simulink library "lib_fuel_converter3"  (Simulink 4.1.1)
values from neighbouring files (symbols this model uses):
  logFlag = 1    [advSACompMaskInit.m]    (also in advSACompMaskInitR13.m)
undefined symbols (not defined in the file or in its folder): air_cp, amb_tmp, cyc_mph, ex_gas_cp, fc_acc_mass, fc_base_mass, fc_c2i_th_cond, fc_c_init_tmp, fc_cl2h_eff, fc_CO2_to_FUELgps, fc_cold, fc_cold_tmp, fc_cp, fc_ct_trq, fc_emisv, fc_ext_sarea, fc_fuel_den, fc_fuel_lhv, fc_h2x_th_cond, fc_h_air_flow, fc_h_cp, fc_h_init_tmp, fc_hood_emisv, fc_hood_sarea, fc_i2x_th_cond, fc_i_init_tmp, fc_inertia, fc_map_spd, fc_map_trq, fc_max_trq, fc_nn_model_name, fc_pwr_scale, fc_spd_scale, fc_trq_scale, fc_tstat, fc_x_init_tmp, fd_ratio, gb_num_init, gb_ratio, generalName, pow, vc_idle_bool, vc_idle_spd, vc_key_on, veh_glider_mass, wh_radius
libraries: lib_fuel_converter3 x4, lib_etc x4, lib_fuel_converter x2, lib_fuel_converter2 x1
(part 7 of 9)

== system lib_fuel_converter3/fuel converter <fc> no fuel at negative torque/IC Engine Model  &  Interface/ic engine model/requested power and energy ==
  trq : Inport  Port=1  LatchInput=off
  spd : Inport  Port=2  LatchInput=off
  Integrator : Integrator  ExternalReset=none  InitialConditionSource=internal  InitialCondition=0  LimitOutput=off  UpperSaturationLimit=inf  LowerSaturationLimit=-inf  ShowSaturationPort=off  ShowStatePort=off  AbsoluteTolerance=auto
  J : Subsystem  TreatAsAtomicUnit=on  mask(enhancedToWorkspace){generalName=generalName, specificName=energy_r, logFlag=logFlag}
      mask prompts: generalName "General Name [char-evaluated]"; specificName "Specific Name [char-literal]"; logFlag "Enable flag (1=on,0=off)"
      mask help: A wrapper for the Simulink "To Workspace" block that allows you to evaluate the name of the variable to log to workspace. This is useful to avoid the double logging errors that occur when you pull in two library models that attempt to log to the same variable.
      mask init:
      | enhancedToWsMaker
      settings: CopyFcn=breakLinkCopyFcn  ParentCloseFcn=breakLinkParCloseFcn  RTWFcnNameOpts=Auto  RTWFileNameOpts=Auto
      mask Help:
      | <h2>Enhanced To Workspace Block</h2>
      | <h3>Parameters</h3>
      | <UL>
      | <li><b>General Name:</b> This is the more general name of the variable. Variables are saved to the workspace as <i>generalName_specificName</i>. Note that this is an evaluated variable. If you would like to type in the value directly, it must be surrounded with single quotes. Otherwise you can input the name of a variable containing a char string.</li>
      | <li><b>Specific Name:</b> This is the specific name of the variable. Note that this is input as a char literal (i.e., you don't need quotes).</li>
      | <li><b>Enable Flag:</b> This flag should have the value of 0 or 1. If 0, the variable will not be logged to the workspace. If 1, the variable will be logged. This is done so that variable logging can be turned off to improve speed.</li>
      | </ul>
      | <h3>Overview</h3>
      | <p>The enhanced to workspace block was put together to allow one to dynamically resolve variable names at run time in simulink. This is most powerful when used in conjunction with a masked subsystem to allow multiple instances of that masked subsytem to be used in the same model. The strategy is to set the generalName in the block mask which will allow the block to change the general name for all variable logging on the fly.
      | <h3>Helper Files</h3>
      | <p>Three m-files are required by the enhancedToWorkspace block. These files are located in the &lt; ADVISOR root &gt;/GUI directory :
      | <ul>
      | <li><i>enhancedToWsMaker.m</i> This file runs the mask initialization for the block</li>
      | <li><i>breakLinkCopyFcn.m</i> This file is used by the block callback when the simulink block is copied. It is necessary to break the link to the enhancedToWorkspace similar to the To Workspace block in order for it to be able to configure itself. (Try copying simulink's To Workspace block--it is impossible to make a link)</li>
      | <li><i>breakLinkParCloseFcn.m</i> This file is similar to the breakLinkCopyFcn and is used when a parent system is closed</li>
      | </ul>
      | <hr>
      | 
      | <p>Created 2003-Jan-21, Michael Patrick O'Keefe, NREL</p>
      | 
      | <!--
      | <VARDEF>
      | <H3>var_name</H3>
      | <UL>
      | <LI><B>data type</B> data type here</LI>
      | <LI><B>units</B> units here</LI>
      | <LI><B>vehicle type</B> vehicle type here</LI>
      | <LI><B>description</B> description here</LI>
      | </UL>
      | </VARDEF>
      | -->
      mask Display: disp([generalName,'_',specificName])
  Product : Product  Inputs=2  Multiplication=Element-wise(.*)  SaturateOnIntegerOverflow=on
  hp : Subsystem  TreatAsAtomicUnit=on  mask(enhancedToWorkspace){generalName=generalName, specificName=pwr_r_hp, logFlag=logFlag}
      mask prompts: generalName "General Name [char-evaluated]"; specificName "Specific Name [char-literal]"; logFlag "Enable flag (1=on,0=off)"
      mask help: A wrapper for the Simulink "To Workspace" block that allows you to evaluate the name of the variable to log to workspace. This is useful to avoid the double logging errors that occur when you pull in two library models that attempt to log to the same variable.
      mask init:
      | enhancedToWsMaker
      settings: CopyFcn=breakLinkCopyFcn  ParentCloseFcn=breakLinkParCloseFcn  RTWFcnNameOpts=Auto  RTWFileNameOpts=Auto
      mask Help:
      | <h2>Enhanced To Workspace Block</h2>
      | <h3>Parameters</h3>
      | <UL>
      | <li><b>General Name:</b> This is the more general name of the variable. Variables are saved to the workspace as <i>generalName_specificName</i>. Note that this is an evaluated variable. If you would like to type in the value directly, it must be surrounded with single quotes. Otherwise you can input the name of a variable containing a char string.</li>
      | <li><b>Specific Name:</b> This is the specific name of the variable. Note that this is input as a char literal (i.e., you don't need quotes).</li>
      | <li><b>Enable Flag:</b> This flag should have the value of 0 or 1. If 0, the variable will not be logged to the workspace. If 1, the variable will be logged. This is done so that variable logging can be turned off to improve speed.</li>
      | </ul>
      | <h3>Overview</h3>
      | <p>The enhanced to workspace block was put together to allow one to dynamically resolve variable names at run time in simulink. This is most powerful when used in conjunction with a masked subsystem to allow multiple instances of that masked subsytem to be used in the same model. The strategy is to set the generalName in the block mask which will allow the block to change the general name for all variable logging on the fly.
      | <h3>Helper Files</h3>
      | <p>Three m-files are required by the enhancedToWorkspace block. These files are located in the &lt; ADVISOR root &gt;/GUI directory :
      | <ul>
      | <li><i>enhancedToWsMaker.m</i> This file runs the mask initialization for the block</li>
      | <li><i>breakLinkCopyFcn.m</i> This file is used by the block callback when the simulink block is copied. It is necessary to break the link to the enhancedToWorkspace similar to the To Workspace block in order for it to be able to configure itself. (Try copying simulink's To Workspace block--it is impossible to make a link)</li>
      | <li><i>breakLinkParCloseFcn.m</i> This file is similar to the breakLinkCopyFcn and is used when a parent system is closed</li>
      | </ul>
      | <hr>
      | 
      | <p>Created 2003-Jan-21, Michael Patrick O'Keefe, NREL</p>
      | 
      | <!--
      | <VARDEF>
      | <H3>var_name</H3>
      | <UL>
      | <LI><B>data type</B> data type here</LI>
      | <LI><B>units</B> units here</LI>
      | <LI><B>vehicle type</B> vehicle type here</LI>
      | <LI><B>description</B> description here</LI>
      | </UL>
      | </VARDEF>
      | -->
      mask Display: disp([generalName,'_',specificName])
  "w -> hp" : Gain  Gain=0.001341022  Multiplication=Element-wise(K.*u)  SaturateOnIntegerOverflow=on
  watts : Subsystem  TreatAsAtomicUnit=on  mask(enhancedToWorkspace){generalName=generalName, specificName=pwr_r, logFlag=logFlag}
      mask prompts: generalName "General Name [char-evaluated]"; specificName "Specific Name [char-literal]"; logFlag "Enable flag (1=on,0=off)"
      mask help: A wrapper for the Simulink "To Workspace" block that allows you to evaluate the name of the variable to log to workspace. This is useful to avoid the double logging errors that occur when you pull in two library models that attempt to log to the same variable.
      mask init:
      | enhancedToWsMaker
      settings: CopyFcn=breakLinkCopyFcn  ParentCloseFcn=breakLinkParCloseFcn  RTWFcnNameOpts=Auto  RTWFileNameOpts=Auto
      mask Help:
      | <h2>Enhanced To Workspace Block</h2>
      | <h3>Parameters</h3>
      | <UL>
      | <li><b>General Name:</b> This is the more general name of the variable. Variables are saved to the workspace as <i>generalName_specificName</i>. Note that this is an evaluated variable. If you would like to type in the value directly, it must be surrounded with single quotes. Otherwise you can input the name of a variable containing a char string.</li>
      | <li><b>Specific Name:</b> This is the specific name of the variable. Note that this is input as a char literal (i.e., you don't need quotes).</li>
      | <li><b>Enable Flag:</b> This flag should have the value of 0 or 1. If 0, the variable will not be logged to the workspace. If 1, the variable will be logged. This is done so that variable logging can be turned off to improve speed.</li>
      | </ul>
      | <h3>Overview</h3>
      | <p>The enhanced to workspace block was put together to allow one to dynamically resolve variable names at run time in simulink. This is most powerful when used in conjunction with a masked subsystem to allow multiple instances of that masked subsytem to be used in the same model. The strategy is to set the generalName in the block mask which will allow the block to change the general name for all variable logging on the fly.
      | <h3>Helper Files</h3>
      | <p>Three m-files are required by the enhancedToWorkspace block. These files are located in the &lt; ADVISOR root &gt;/GUI directory :
      | <ul>
      | <li><i>enhancedToWsMaker.m</i> This file runs the mask initialization for the block</li>
      | <li><i>breakLinkCopyFcn.m</i> This file is used by the block callback when the simulink block is copied. It is necessary to break the link to the enhancedToWorkspace similar to the To Workspace block in order for it to be able to configure itself. (Try copying simulink's To Workspace block--it is impossible to make a link)</li>
      | <li><i>breakLinkParCloseFcn.m</i> This file is similar to the breakLinkCopyFcn and is used when a parent system is closed</li>
      | </ul>
      | <hr>
      | 
      | <p>Created 2003-Jan-21, Michael Patrick O'Keefe, NREL</p>
      | 
      | <!--
      | <VARDEF>
      | <H3>var_name</H3>
      | <UL>
      | <LI><B>data type</B> data type here</LI>
      | <LI><B>units</B> units here</LI>
      | <LI><B>vehicle type</B> vehicle type here</LI>
      | <LI><B>description</B> description here</LI>
      | </UL>
      | </VARDEF>
      | -->
      mask Display: disp([generalName,'_',specificName])
  wires:
  "w -> hp"/1 -> hp/1(In1)
  Product/1 -> "w -> hp"/1, Integrator/1, watts/1(In1)
  Integrator/1 -> J/1(In1)
  trq/1 -> Product/1
  spd/1 -> Product/2

== system lib_fuel_converter3/Fuel Converter Control/Fuel Converter Control conventional ic engine/conventional IC engine/Fuel Converter Control/key_on ==
  Clock : Clock
      settings: DisplayTime=off  Decimation=10
  Fcn1 : Fcn  Expr=rem(u[1],period)
  Look-Up Table : Lookup  InputValues=t  OutputValues=y
  out_1 : Outport  Port=1  InitialOutput=0
  wires:
  Fcn1/1 -> Look-Up Table/1
  Clock/1 -> Fcn1/1
  Look-Up Table/1 -> out_1/1

== system lib_fuel_converter3/configurable subsystems/fuel use and EO emis/fc temp/fc mass heat flow/Block NOTES ==
  note: FUEL CONVERTER MASS HEAT LOSS
      | This block models the heat loss from a fuel converter (such as an IC engine).
      | Convection (as a function of vehicle speed), radiation, and conduction effects are included.
      | Engine cylinder (c), interior (i), exterior (x) and hood (h)
      | heat flows are estimated based on the temperatures from the previous iteration.

== system lib_fuel_converter3/configurable subsystems/fuel use and EO emis/fc temp/old fc coolant  temp. (C)/Block NOTES ==
  note: This block computes engine coolant temperature,
      | assuming that it asymptotically approaches its maximum
      | temperature when the engine is on, and asymptotically
      | approaches the ambient temperature when the engine
      | is off.  Temperatue rise rate is assumed to be a function
      | only of current engine coolant temperature, and the fall
      | rate is also a function of vehicle speed and ambient temperature.
      | There is no dependence on engine load or speed.

== system lib_fuel_converter3/configurable subsystems/fuel use and EO emis/fc temp correct/fc temp correct Constant Correction Factors (Equation Based)/Block NOTES ==
  note: This block determines actual fuel use and engine-out emissions
      | given the fully hot values and the engine coolant temperature.
      | The correlations used here were developed at NREL using
      | Hot and Cold Engine data collected
      | at Oak Ridge National Laboratory.

== system lib_fuel_converter3/configurable subsystems/fuel use and EO emis/fc temp correct/fc temp correct Variable Correction Factors (Map Based)/CO factor cold-to-hot ==
  x0 : Inport  Port=1  LatchInput=off
  y0 : Inport  Port=2  LatchInput=off
  Mux : Mux  Inputs=2
      settings: DisplayOption=none
  S-function : S-Function  FunctionName=sftable2  Parameters=xindex, yindex, table  PortCounts=[]  SFunctionModules=''
  table out : Outport  Port=1  InitialOutput=0
  wires:
  y0/1 -> Mux/2
  S-function/1 -> table out/1
  x0/1 -> Mux/1
  Mux/1 -> S-function/1

== system lib_fuel_converter3/configurable subsystems/fuel use and EO emis/fc temp correct/fc temp correct Variable Correction Factors (Map Based)/HC factor cold-to-hot ==
  x0 : Inport  Port=1  LatchInput=off
  y0 : Inport  Port=2  LatchInput=off
  Mux : Mux  Inputs=2
      settings: DisplayOption=none
  S-function : S-Function  FunctionName=sftable2  Parameters=xindex, yindex, table  PortCounts=[]  SFunctionModules=''
  table out : Outport  Port=1  InitialOutput=0
  wires:
  y0/1 -> Mux/2
  S-function/1 -> table out/1
  x0/1 -> Mux/1
  Mux/1 -> S-function/1

== system lib_fuel_converter3/configurable subsystems/fuel use and EO emis/fc temp correct/fc temp correct Variable Correction Factors (Map Based)/NOx factor cold-to-hot ==
  x0 : Inport  Port=1  LatchInput=off
  y0 : Inport  Port=2  LatchInput=off
  Mux : Mux  Inputs=2
      settings: DisplayOption=none
  S-function : S-Function  FunctionName=sftable2  Parameters=xindex, yindex, table  PortCounts=[]  SFunctionModules=''
  table out : Outport  Port=1  InitialOutput=0
  wires:
  y0/1 -> Mux/2
  S-function/1 -> table out/1
  x0/1 -> Mux/1
  Mux/1 -> S-function/1

== system lib_fuel_converter3/configurable subsystems/fuel use and EO emis/fc temp correct/fc temp correct Variable Correction Factors (Map Based)/PM factor cold-to-hot ==
  x0 : Inport  Port=1  LatchInput=off
  y0 : Inport  Port=2  LatchInput=off
  Mux : Mux  Inputs=2
      settings: DisplayOption=none
  S-function : S-Function  FunctionName=sftable2  Parameters=xindex, yindex, table  PortCounts=[]  SFunctionModules=''
  table out : Outport  Port=1  InitialOutput=0
  wires:
  y0/1 -> Mux/2
  S-function/1 -> table out/1
  x0/1 -> Mux/1
  Mux/1 -> S-function/1

== system lib_fuel_converter3/configurable subsystems/fuel use and EO emis/fc temp correct/fc temp correct Variable Correction Factors (Map Based)/fuel factor cold-to-hot ==
  x0 : Inport  Port=1  LatchInput=off
  y0 : Inport  Port=2  LatchInput=off
  Mux : Mux  Inputs=2
      settings: DisplayOption=none
  S-function : S-Function  FunctionName=sftable2  Parameters=xindex, yindex, table  PortCounts=[]  SFunctionModules=''
  table out : Outport  Port=1  InitialOutput=0
  wires:
  y0/1 -> Mux/2
  S-function/1 -> table out/1
  x0/1 -> Mux/1
  Mux/1 -> S-function/1

== system lib_fuel_converter3/configurable subsystems/fuel use and EO emis Neural Network Model/fc temp/fc mass heat flow/Block NOTES ==
  note: FUEL CONVERTER MASS HEAT LOSS
      | This block models the heat loss from a fuel converter (such as an IC engine).
      | Convection (as a function of vehicle speed), radiation, and conduction effects are included.
      | Engine cylinder (c), interior (i), exterior (x) and hood (h)
      | heat flows are estimated based on the temperatures from the previous iteration.

== system lib_fuel_converter3/configurable subsystems/fuel use and EO emis Neural Network Model/fc temp/old fc coolant  temp. (C)/Block NOTES ==
  note: This block computes engine coolant temperature,
      | assuming that it asymptotically approaches its maximum
      | temperature when the engine is on, and asymptotically
      | approaches the ambient temperature when the engine
      | is off.  Temperatue rise rate is assumed to be a function
      | only of current engine coolant temperature, and the fall
      | rate is also a function of vehicle speed and ambient temperature.
      | There is no dependence on engine load or speed.

== system lib_fuel_converter3/configurable subsystems/fuel use and EO emis Neural Network Model/fc temp correct/fc temp correct Constant Correction Factors (Equation Based)/Block NOTES ==
  note: This block determines actual fuel use and engine-out emissions
      | given the fully hot values and the engine coolant temperature.
      | The correlations used here were developed at NREL using
      | Hot and Cold Engine data collected
      | at Oak Ridge National Laboratory.

== system lib_fuel_converter3/configurable subsystems/fuel use and EO emis Neural Network Model/fc temp correct/fc temp correct Variable Correction Factors (Map Based)/CO factor cold-to-hot ==
  x0 : Inport  Port=1  LatchInput=off
  y0 : Inport  Port=2  LatchInput=off
  Mux : Mux  Inputs=2
      settings: DisplayOption=none
  S-function : S-Function  FunctionName=sftable2  Parameters=xindex, yindex, table  PortCounts=[]  SFunctionModules=''
  table out : Outport  Port=1  InitialOutput=0
  wires:
  y0/1 -> Mux/2
  S-function/1 -> table out/1
  x0/1 -> Mux/1
  Mux/1 -> S-function/1

== system lib_fuel_converter3/configurable subsystems/fuel use and EO emis Neural Network Model/fc temp correct/fc temp correct Variable Correction Factors (Map Based)/HC factor cold-to-hot ==
  x0 : Inport  Port=1  LatchInput=off
  y0 : Inport  Port=2  LatchInput=off
  Mux : Mux  Inputs=2
      settings: DisplayOption=none
  S-function : S-Function  FunctionName=sftable2  Parameters=xindex, yindex, table  PortCounts=[]  SFunctionModules=''
  table out : Outport  Port=1  InitialOutput=0
  wires:
  y0/1 -> Mux/2
  S-function/1 -> table out/1
  x0/1 -> Mux/1
  Mux/1 -> S-function/1

== system lib_fuel_converter3/configurable subsystems/fuel use and EO emis Neural Network Model/fc temp correct/fc temp correct Variable Correction Factors (Map Based)/NOx factor cold-to-hot ==
  x0 : Inport  Port=1  LatchInput=off
  y0 : Inport  Port=2  LatchInput=off
  Mux : Mux  Inputs=2
      settings: DisplayOption=none
  S-function : S-Function  FunctionName=sftable2  Parameters=xindex, yindex, table  PortCounts=[]  SFunctionModules=''
  table out : Outport  Port=1  InitialOutput=0
  wires:
  y0/1 -> Mux/2
  S-function/1 -> table out/1
  x0/1 -> Mux/1
  Mux/1 -> S-function/1

== system lib_fuel_converter3/configurable subsystems/fuel use and EO emis Neural Network Model/fc temp correct/fc temp correct Variable Correction Factors (Map Based)/PM factor cold-to-hot ==
  x0 : Inport  Port=1  LatchInput=off
  y0 : Inport  Port=2  LatchInput=off
  Mux : Mux  Inputs=2
      settings: DisplayOption=none
  S-function : S-Function  FunctionName=sftable2  Parameters=xindex, yindex, table  PortCounts=[]  SFunctionModules=''
  table out : Outport  Port=1  InitialOutput=0
  wires:
  y0/1 -> Mux/2
  S-function/1 -> table out/1
  x0/1 -> Mux/1
  Mux/1 -> S-function/1

== system lib_fuel_converter3/configurable subsystems/fuel use and EO emis Neural Network Model/fc temp correct/fc temp correct Variable Correction Factors (Map Based)/fuel factor cold-to-hot ==
  x0 : Inport  Port=1  LatchInput=off
  y0 : Inport  Port=2  LatchInput=off
  Mux : Mux  Inputs=2
      settings: DisplayOption=none
  S-function : S-Function  FunctionName=sftable2  Parameters=xindex, yindex, table  PortCounts=[]  SFunctionModules=''
  table out : Outport  Port=1  InitialOutput=0
  wires:
  y0/1 -> Mux/2
  S-function/1 -> table out/1
  x0/1 -> Mux/1
  Mux/1 -> S-function/1

== system lib_fuel_converter3/fuel converter  <fc> for series/Model & Interface/model/providing trq (+ive or -ive)/effect of inertia (Nm) ==
  note: if initial speed is >0 and it is the
      | first time step ignore inertial loads
      | tm:2/6/01
  req'd spd (rad/s) : Inport  Port=1  LatchInput=off
  prev spd : Inport  Port=2  LatchInput=off
  Clock : Clock
      settings: DisplayTime=off  Decimation=10
  Constant : Constant  Value=fc_inertia
  Constant1 : Constant  Value=cyc_mph(1,2)
  Logical Operator : Logic  Operator=NAND  Inputs=2
  Logical Operator1 : Logic  Operator=NOT  Inputs=2
  Memory : Memory  X0=-0.1  InheritSampleTime=off
      settings: RTWStateStorageClass=Auto
  Memory1 : Memory  X0=0  InheritSampleTime=off
      settings: RTWStateStorageClass=Auto
  Product1 : Product  Inputs=**/*  Multiplication=Element-wise(.*)  SaturateOnIntegerOverflow=on
  Sum : Sum  Inputs=+-  SaturateOnIntegerOverflow=on
  Sum1 : Sum  Inputs=+-  SaturateOnIntegerOverflow=on
  (Nm) : Outport  Port=1  InitialOutput=0
  wires:
  Logical Operator1/1 -> Logical Operator/2
  Memory1/1 -> Logical Operator1/1
  Constant1/1 -> Logical Operator/1
  Logical Operator/1 -> Product1/4
  Sum/1 -> Product1/2
  Sum1/1 -> Product1/3
  req'd spd (rad/s)/1 -> Sum/1
  prev spd/1 -> Sum/2
  Product1/1 -> (Nm)/1
  Memory/1 -> Sum1/2
  Clock/1 -> Memory1/1, Memory/1, Sum1/1
  Constant/1 -> Product1/1

== system lib_fuel_converter3/fuel converter  <fc> for series/Model & Interface/model/providing trq (+ive or -ive)/enforce engine limits ==
  req'd engine trq (Nm) : Inport  Port=1  LatchInput=off
  req'd engine spd (rad/s) : Inport  Port=2  LatchInput=off
  Block NOTES : Subsystem
      settings: RTWFcnNameOpts=Auto  RTWFileNameOpts=Auto
      mask Display: disp('Block\nNOTES')
  MinMax : MinMax  Function=min  Inputs=2
  MinMax1 : MinMax  Function=max  Inputs=2
  Relational Operator : RelationalOperator  Operator=~=
  Saturation : Saturate  UpperLimit=max(fc_map_spd)*fc_spd_scale  LowerLimit=0  LinearizeAsGain=on
  T_closed throttle : lib_fuel_converter/fuel converter  <fc> for series/providing trq (+ive or -ive)/enforce engine limits/T_closed throttle
      settings: RTWFcnNameOpts=Auto  RTWFileNameOpts=Auto
  T_max : Subsystem
      settings: RTWFcnNameOpts=Auto  RTWFileNameOpts=Auto
  clutch disengaged1 : RelationalOperator  Operator=~=
  limited engine brake trq (Nm) : Outport  Port=1
  limited engine spd (rad/s) : Outport  Port=2
  tag scope: fc_spd_limited=scoped, fc_trq_limited=scoped
  wires:
  Relational Operator/1 -> [fc_spd_limited]
  MinMax/1 -> MinMax1/1
  T_max/1(T_max) -> MinMax/2
  clutch disengaged1/1 -> [fc_trq_limited]
  MinMax1/1 -> limited engine brake trq (Nm)/1, clutch disengaged1/2
  req'd engine trq (Nm)/1 -> MinMax/1, clutch disengaged1/1
  Saturation/1 -> T_closed throttle/1, T_max/1(w_APU), limited engine spd (rad/s)/1, Relational Operator/2
  req'd engine spd (rad/s)/1 -> Saturation/1, Relational Operator/1
  T_closed throttle/1 -> MinMax1/2

== system lib_fuel_converter3/fuel converter  <fc> for series/Model & Interface/model/spinning up or spinning down/T_closed throttle ==
  w_APU : Inport  Port=1  LatchInput=off
  Saturation : Saturate  UpperLimit=max(fc_map_spd)*fc_spd_scale  LowerLimit=min(fc_map_spd)*fc_spd_scale  LinearizeAsGain=on
  ctt lookup : Lookup  InputValues=fc_map_spd*fc_spd_scale  OutputValues=fc_ct_trq*fc_trq_scale
  T_closed throttle : Outport  Port=1  InitialOutput=0
  wires:
  w_APU/1 -> Saturation/1
  Saturation/1 -> ctt lookup/1
  ctt lookup/1 -> T_closed throttle/1

== system lib_fuel_converter3/fuel converter  <fc> for series/Model & Interface/model/spinning up or spinning down/T_max ==
  w_APU : Inport  Port=1  LatchInput=off
  Saturation1 : Saturate  UpperLimit=max(fc_map_spd)*fc_spd_scale  LowerLimit=min(fc_map_spd)*fc_spd_scale  LinearizeAsGain=on
  max_torque lookup : Lookup  InputValues=fc_map_spd*fc_spd_scale  OutputValues=fc_max_trq*fc_trq_scale
  T_max : Outport  Port=1  InitialOutput=0
  wires:
  max_torque lookup/1 -> T_max/1
  w_APU/1 -> Saturation1/1
  Saturation1/1 -> max_torque lookup/1

== system lib_fuel_converter3/fuel converter  <fc> for series/Model & Interface/model/spinning up or spinning down/dt ==
  Clock : Clock
      settings: DisplayTime=off  Decimation=10
  Memory1 : Memory  X0=-0.1  InheritSampleTime=off
      settings: RTWStateStorageClass=Auto
  Sum1 : Sum  Inputs=+-  SaturateOnIntegerOverflow=on
  out_1 : Outport  Port=1  InitialOutput=0
  wires:
  Sum1/1 -> out_1/1
  Memory1/1 -> Sum1/2
  Clock/1 -> Memory1/1, Sum1/1

== system lib_fuel_converter3/fuel converter  <fc> for series/Model & Interface/model/spinning up or spinning down/effect of inertia (Nm) ==
  note: if initial speed is >0 and it is the
      | first time step ignore inertial loads
      | tm:2/6/01
  req'd spd (rad/s) : Inport  Port=1  LatchInput=off
  prev spd : Inport  Port=2  LatchInput=off
  Clock : Clock
      settings: DisplayTime=off  Decimation=10
  Constant : Constant  Value=fc_inertia
  Constant1 : Constant  Value=cyc_mph(1,2)
  Logical Operator : Logic  Operator=NAND  Inputs=2
  Logical Operator1 : Logic  Operator=NOT  Inputs=2
  Memory : Memory  X0=-0.1  InheritSampleTime=off
      settings: RTWStateStorageClass=Auto
  Memory1 : Memory  X0=0  InheritSampleTime=off
      settings: RTWStateStorageClass=Auto
  Product1 : Product  Inputs=**/*  Multiplication=Element-wise(.*)  SaturateOnIntegerOverflow=on
  Sum : Sum  Inputs=+-  SaturateOnIntegerOverflow=on
  Sum1 : Sum  Inputs=+-  SaturateOnIntegerOverflow=on
  (Nm) : Outport  Port=1  InitialOutput=0
  wires:
  Constant/1 -> Product1/1
  Clock/1 -> Sum1/1, Memory/1, Memory1/1
  Memory/1 -> Sum1/2
  Product1/1 -> (Nm)/1
  prev spd/1 -> Sum/2
  req'd spd (rad/s)/1 -> Sum/1
  Sum1/1 -> Product1/3
  Sum/1 -> Product1/2
  Logical Operator/1 -> Product1/4
  Constant1/1 -> Logical Operator/1
  Memory1/1 -> Logical Operator1/1
  Logical Operator1/1 -> Logical Operator/2

== system lib_fuel_converter3/fuel converter  <fc> for series/Model & Interface/model/spinning up or spinning down/just started spin-down/spin-up ==
  state : Inport  Port=1  LatchInput=off
  Logical Operator : Logic  Operator=AND  Inputs=2
  Logical Operator1 : Logic  Operator=NOT  Inputs=1
  Memory1 : Memory  X0=(cyc_mph(1,2)==0)  InheritSampleTime=off
      settings: RTWStateStorageClass=Auto
  trigger : Outport  Port=1  InitialOutput=0
  wires:
  state/1 -> Memory1/1, Logical Operator/1
  Logical Operator/1 -> trigger/1
  Logical Operator1/1 -> Logical Operator/2
  Memory1/1 -> Logical Operator1/1

== system lib_fuel_converter3/fuel converter  <fc> for series/Model & Interface/model/spinning up or spinning down/no-lag Reset Integrator ==
  in_1 : Inport  Port=1  LatchInput=off
  in_2 : Inport  Port=2  LatchInput=off
  in_3 : Inport  Port=3  LatchInput=off
  Constant : Constant  Value=0
  Memory : Memory  Orientation=left  X0=initval  InheritSampleTime=off
      settings: RTWStateStorageClass=Auto
  Product : Product  Inputs=2  Multiplication=Element-wise(.*)  SaturateOnIntegerOverflow=on
  Sum : Sum  Inputs=++  SaturateOnIntegerOverflow=on
  Switch : Switch  Threshold=eps
  dt : lib_fuel_converter/fuel converter  <fc> for series/spinning up or spinning down/no-lag Reset Integrator/dt  Orientation=down
      settings: RTWFcnNameOpts=Auto  RTWFileNameOpts=Auto
  in_2==0 : RelationalOperator  Operator===
  out_1 : Outport  Port=1  InitialOutput=0
  wires:
  Constant/1 -> in_2==0/2
  in_2==0/1 -> Switch/2
  Switch/1 -> Memory/1, out_1/1
  Sum/1 -> Switch/1
  Memory/1 -> Sum/1
  Product/1 -> Sum/2
  dt/1 -> Product/1
  in_1/1 -> Product/2
  in_2/1 -> in_2==0/1
  in_3/1 -> Switch/3

== system lib_fuel_converter3/fuel converter <fc>/IC Engine Model  &  Interface/ic engine model/engine speed estimator/Block NOTES ==
  note: If the clutch is engaged and the trace was missed in the previous time step:
      | The estimated engine speed for the current time step is the actual engine
      | speed from the previous time step.
      |
      | If the clutch is disengaged and the speed is commanded to increase (spin up):
      | The engine speed is the lesser of the commanded speed and the maximum
      | speed attainable given the engine capability.
      |
      | If the clutch is disengaged at the speed is commanded to decrease (spin down):
      | The engine speed is computed by integrating with respect to time the ratio of
      |  closed-throttle torque to engine inertia.
      |
      | Otherwise:
      | The engine speed is equal to the speed command, but no greater than the
      | engine's maximum speed nor less than the engine's idle speed (if the engine is on.)

== system lib_fuel_converter3/fuel converter <fc>/IC Engine Model  &  Interface/ic engine model/engine speed estimator/dt ==
  Clock : Clock
      settings: DisplayTime=off  Decimation=10
  Memory1 : Memory  X0=-0.1  InheritSampleTime=off
      settings: RTWStateStorageClass=Auto
  Sum1 : Sum  Inputs=+-  SaturateOnIntegerOverflow=on
  out_1 : Outport  Port=1  InitialOutput=0
  wires:
  Sum1/1 -> out_1/1
  Memory1/1 -> Sum1/2
  Clock/1 -> Memory1/1, Sum1/1

== system lib_fuel_converter3/fuel converter <fc>/IC Engine Model  &  Interface/ic engine model/engine speed estimator/effect of inertia (Nm) ==
  req'd spd (rad/s) : Inport  Port=1  LatchInput=off
  prev spd : Inport  Port=2  LatchInput=off
  Clock : Clock
      settings: DisplayTime=off  Decimation=10
  Constant : Constant  Value=fc_inertia
  Memory : Memory  X0=-0.1  InheritSampleTime=off
      settings: RTWStateStorageClass=Auto
  Product1 : Product  Inputs=**/  Multiplication=Element-wise(.*)  SaturateOnIntegerOverflow=on
  Sum : Sum  Inputs=+-  SaturateOnIntegerOverflow=on
  Sum1 : Sum  Inputs=+-  SaturateOnIntegerOverflow=on
  (Nm) : Outport  Port=1  InitialOutput=0
  wires:
  Sum/1 -> Product1/2
  Sum1/1 -> Product1/3
  req'd spd (rad/s)/1 -> Sum/1
  prev spd/1 -> Sum/2
  Product1/1 -> (Nm)/1
  Memory/1 -> Sum1/2
  Clock/1 -> Memory/1, Sum1/1
  Constant/1 -> Product1/1

== system lib_fuel_converter3/fuel converter <fc>/IC Engine Model  &  Interface/ic engine model/engine speed estimator/just started spin-down/spin-up ==
  state : Inport  Port=1  LatchInput=off
  Logical Operator : Logic  Operator=AND  Inputs=2
  Logical Operator1 : Logic  Operator=NOT  Inputs=1
  Memory1 : Memory  X0=1  InheritSampleTime=off
      settings: RTWStateStorageClass=Auto
  trigger : Outport  Port=1  InitialOutput=0
  wires:
  Memory1/1 -> Logical Operator1/1
  Logical Operator1/1 -> Logical Operator/2
  Logical Operator/1 -> trigger/1
  state/1 -> Logical Operator/1, Memory1/1

== system lib_fuel_converter3/fuel converter <fc>/IC Engine Model  &  Interface/ic engine model/engine speed estimator/no-lag Reset Integrator ==
  in_1 : Inport  Port=1  LatchInput=off
  in_2 : Inport  Port=2  LatchInput=off
  in_3 : Inport  Port=3  LatchInput=off
  Constant : Constant  Value=0
  Memory : Memory  Orientation=left  X0=initval  InheritSampleTime=off
      settings: RTWStateStorageClass=Auto
  Product : Product  Inputs=2  Multiplication=Element-wise(.*)  SaturateOnIntegerOverflow=on
  Sum : Sum  Inputs=++  SaturateOnIntegerOverflow=on
  Switch : Switch  Threshold=eps
  dt : Subsystem  Orientation=down
      settings: RTWFcnNameOpts=Auto  RTWFileNameOpts=Auto
  in_2==0 : RelationalOperator  Operator===
  out_1 : Outport  Port=1  InitialOutput=0
  wires:
  in_3/1 -> Switch/3
  in_2/1 -> in_2==0/1
  in_1/1 -> Product/2
  dt/1(out_1) -> Product/1
  Product/1 -> Sum/2
  Memory/1 -> Sum/1
  Sum/1 -> Switch/1
  Switch/1 -> out_1/1, Memory/1
  in_2==0/1 -> Switch/2
  Constant/1 -> in_2==0/2

== system lib_fuel_converter3/fuel converter <fc>/IC Engine Model  &  Interface/ic engine model/engine torque/Block NOTES ==
  note: If the engine is not spinning down with the clutch disengaged:
      | 1.  Engine brake (aka map) torque is given by the required shaft
      | torque plus enough torque to accelerate the engine's rotating
      | parts as commanded and torque to power the accessories,
      | subject to the engine's torque limits at the current speed.
      | 2.  Shaft torque is engine brake torque less the effects of inertia
      | and accessories.
      |
      | If the engine is spinning down:
      | 1.  Engine brake/map torque is the closed-throttle torque.
      | 2.  Shaft torque is zero.

== system lib_fuel_converter3/fuel converter <fc>/IC Engine Model  &  Interface/ic engine model/engine torque/T_closed throttle ==
  w_APU : Inport  Port=1  LatchInput=off
  Saturation : Saturate  UpperLimit=max(fc_map_spd)*fc_spd_scale  LowerLimit=min(fc_map_spd)*fc_spd_scale  LinearizeAsGain=on
  ctt lookup : Lookup  InputValues=fc_map_spd*fc_spd_scale  OutputValues=fc_ct_trq*fc_trq_scale
  T_closed throttle : Outport  Port=1  InitialOutput=0
  wires:
  w_APU/1 -> Saturation/1
  Saturation/1 -> ctt lookup/1
  ctt lookup/1 -> T_closed throttle/1

== system lib_fuel_converter3/fuel converter <fc>/IC Engine Model  &  Interface/ic engine model/engine torque/T_max ==
  w_APU : Inport  Port=1  LatchInput=off
  Saturation1 : Saturate  UpperLimit=max(fc_map_spd)*fc_spd_scale  LowerLimit=min(fc_map_spd)*fc_spd_scale  LinearizeAsGain=on
  max_torque lookup : Lookup  InputValues=fc_map_spd*fc_spd_scale  OutputValues=fc_max_trq*fc_trq_scale
  T_max : Outport  Port=1  InitialOutput=0
  tag scope: engine_speed=scoped
  wires:
  Saturation1/1 -> [engine_speed], max_torque lookup/1
  max_torque lookup/1 -> T_max/1
  w_APU/1 -> Saturation1/1

== system lib_fuel_converter3/fuel converter <fc>/IC Engine Model  &  Interface/ic engine model/engine torque/effect of inertia (Nm) ==
  engine spd (rad/s) : Inport  Port=1  LatchInput=off
  >=0 : Saturate  UpperLimit=inf  LowerLimit=0  LinearizeAsGain=on
  Block NOTES : Subsystem
      settings: RTWFcnNameOpts=Auto  RTWFileNameOpts=Auto
      mask Display: disp('Block\nNOTES')
  Clock : Clock
      settings: DisplayTime=off  Decimation=10
  Constant : Constant  Orientation=left  Value=fc_inertia
  Constant1 : Constant  Value=max(fc_max_trq)*fc_trq_scale
  Constant2 : Constant  Orientation=left  Value=0.01
  Memory : Memory  X0=-0.1  InheritSampleTime=off
      settings: RTWStateStorageClass=Auto
  Memory1 : Memory  X0=vc_idle_spd*vc_key_on(1,2)  InheritSampleTime=off
      settings: RTWStateStorageClass=Auto
  MinMax : MinMax  Function=min  Inputs=2
  Product : Product  Inputs=2  Multiplication=Element-wise(.*)  SaturateOnIntegerOverflow=on
  Product1 : Product  Inputs=*/*  Multiplication=Element-wise(.*)  SaturateOnIntegerOverflow=on
  Relational : RelationalOperator  Operator=>
  Sum : Sum  Inputs=+-  SaturateOnIntegerOverflow=on
  Sum1 : Sum  Inputs=+-  SaturateOnIntegerOverflow=on
  Sum2 : Sum  Inputs=-+  SaturateOnIntegerOverflow=on
  Switch : Switch  Threshold=eps
  engine inertia as a function of total vehicle inertia (generous approximation) : Subsystem  Orientation=down
      settings: RTWFcnNameOpts=Auto  RTWFileNameOpts=Auto
  (Nm) : Outport  Port=1  InitialOutput=0
  wires:
  engine spd (rad/s)/1 -> Sum/1, Memory1/1
  Constant2/1 -> Relational/2
  Sum2/1 -> Relational/1
  >=0/1 -> Switch/1
  Relational/1 -> Switch/2
  Clock/1 -> Sum1/1, Memory/1
  Memory/1 -> Sum1/2
  Constant/1 -> Product1/3
  Sum1/1 -> Product1/2
  Switch/1 -> Product1/1
  [mpha_prev] -> Sum2/1
  [cyc_mph_r_prev] -> Sum2/2
  MinMax/1 -> (Nm)/1
  Product1/1 -> MinMax/2
  engine inertia as a function of total vehicle inertia (generous approximation)/1(Out1) -> Product/1
  Constant1/1 -> Product/2
  Product/1 -> MinMax/1
  Memory1/1 -> Sum/2
  Sum/1 -> Switch/3, >=0/1

== system lib_fuel_converter3/fuel converter <fc> no fuel at negative torque/IC Engine Model  &  Interface/ic engine model/achieved power and energy/J ==
  In1 : Inport  Port=1  LatchInput=off
  To Workspace : ToWorkspace  VariableName=fc_energy_a  SampleTime=-1  SaveFormat=Array
  wires:
  In1/1 -> To Workspace/1

== system lib_fuel_converter3/fuel converter <fc> no fuel at negative torque/IC Engine Model  &  Interface/ic engine model/achieved power and energy/hp ==
  In1 : Inport  Port=1  LatchInput=off
  To Workspace : ToWorkspace  VariableName=fc_pwr_a_hp  SampleTime=-1  SaveFormat=Array
  wires:
  In1/1 -> To Workspace/1

== system lib_fuel_converter3/fuel converter <fc> no fuel at negative torque/IC Engine Model  &  Interface/ic engine model/achieved power and energy/watts ==
  In1 : Inport  Port=1  LatchInput=off
  To Workspace : ToWorkspace  VariableName=fc_pwr_a  SampleTime=-1  SaveFormat=Array
  wires:
  In1/1 -> To Workspace/1

== system lib_fuel_converter3/fuel converter <fc> no fuel at negative torque/IC Engine Model  &  Interface/ic engine model/engine speed estimator/Block NOTES ==
  note: If the clutch is engaged and the trace was missed in the previous time step:
      | The estimated engine speed for the current time step is the actual engine
      | speed from the previous time step.
      |
      | If the clutch is disengaged and the speed is commanded to increase (spin up):
      | The engine speed is the lesser of the commanded speed and the maximum
      | speed attainable given the engine capability.
      |
      | If the clutch is disengaged at the speed is commanded to decrease (spin down):
      | The engine speed is computed by integrating with respect to time the ratio of
      |  closed-throttle torque to engine inertia.
      |
      | Otherwise:
      | The engine speed is equal to the speed command, but no greater than the
      | engine's maximum speed nor less than the engine's idle speed (if the engine is on.)

== system lib_fuel_converter3/fuel converter <fc> no fuel at negative torque/IC Engine Model  &  Interface/ic engine model/engine speed estimator/dt ==
  Clock : Clock
      settings: DisplayTime=off  Decimation=10
  Memory1 : Memory  X0=-0.1  InheritSampleTime=off
      settings: RTWStateStorageClass=Auto
  Sum1 : Sum  Inputs=+-  SaturateOnIntegerOverflow=on
  out_1 : Outport  Port=1  InitialOutput=0
  wires:
  Sum1/1 -> out_1/1
  Memory1/1 -> Sum1/2
  Clock/1 -> Memory1/1, Sum1/1

== system lib_fuel_converter3/fuel converter <fc> no fuel at negative torque/IC Engine Model  &  Interface/ic engine model/engine speed estimator/effect of inertia (Nm) ==
  req'd spd (rad/s) : Inport  Port=1  LatchInput=off
  prev spd : Inport  Port=2  LatchInput=off
  Clock : Clock
      settings: DisplayTime=off  Decimation=10
  Constant : Constant  Value=fc_inertia
  Memory : Memory  X0=-0.1  InheritSampleTime=off
      settings: RTWStateStorageClass=Auto
  Product1 : Product  Inputs=**/  Multiplication=Element-wise(.*)  SaturateOnIntegerOverflow=on
  Sum : Sum  Inputs=+-  SaturateOnIntegerOverflow=on
  Sum1 : Sum  Inputs=+-  SaturateOnIntegerOverflow=on
  (Nm) : Outport  Port=1  InitialOutput=0
  wires:
  Sum/1 -> Product1/2
  Sum1/1 -> Product1/3
  req'd spd (rad/s)/1 -> Sum/1
  prev spd/1 -> Sum/2
  Product1/1 -> (Nm)/1
  Memory/1 -> Sum1/2
  Clock/1 -> Memory/1, Sum1/1
  Constant/1 -> Product1/1

== system lib_fuel_converter3/fuel converter <fc> no fuel at negative torque/IC Engine Model  &  Interface/ic engine model/engine speed estimator/just started spin-down/spin-up ==
  state : Inport  Port=1  LatchInput=off
  Logical Operator : Logic  Operator=AND  Inputs=2
  Logical Operator1 : Logic  Operator=NOT  Inputs=1
  Memory1 : Memory  X0=1  InheritSampleTime=off
      settings: RTWStateStorageClass=Auto
  trigger : Outport  Port=1  InitialOutput=0
  wires:
  Memory1/1 -> Logical Operator1/1
  Logical Operator1/1 -> Logical Operator/2
  Logical Operator/1 -> trigger/1
  state/1 -> Logical Operator/1, Memory1/1

== system lib_fuel_converter3/fuel converter <fc> no fuel at negative torque/IC Engine Model  &  Interface/ic engine model/engine speed estimator/no-lag Reset Integrator ==
  in_1 : Inport  Port=1  LatchInput=off
  in_2 : Inport  Port=2  LatchInput=off
  in_3 : Inport  Port=3  LatchInput=off
  Constant : Constant  Value=0
  Memory : Memory  Orientation=left  X0=initval  InheritSampleTime=off
      settings: RTWStateStorageClass=Auto
  Product : Product  Inputs=2  Multiplication=Element-wise(.*)  SaturateOnIntegerOverflow=on
  Sum : Sum  Inputs=++  SaturateOnIntegerOverflow=on
  Switch : Switch  Threshold=eps
  dt : Subsystem  Orientation=down
      settings: RTWFcnNameOpts=Auto  RTWFileNameOpts=Auto
  in_2==0 : RelationalOperator  Operator===
  out_1 : Outport  Port=1  InitialOutput=0
  wires:
  in_3/1 -> Switch/3
  in_2/1 -> in_2==0/1
  in_1/1 -> Product/2
  dt/1(out_1) -> Product/1
  Product/1 -> Sum/2
  Memory/1 -> Sum/1
  Sum/1 -> Switch/1
  Switch/1 -> out_1/1, Memory/1
  in_2==0/1 -> Switch/2
  Constant/1 -> in_2==0/2

== system lib_fuel_converter3/fuel converter <fc> no fuel at negative torque/IC Engine Model  &  Interface/ic engine model/engine torque/Block NOTES ==
  note: If the engine is not spinning down with the clutch disengaged:
      | 1.  Engine brake (aka map) torque is given by the required shaft
      | torque plus enough torque to accelerate the engine's rotating
      | parts as commanded and torque to power the accessories,
      | subject to the engine's torque limits at the current speed.
      | 2.  Shaft torque is engine brake torque less the effects of inertia
      | and accessories.
      |
      | If the engine is spinning down:
      | 1.  Engine brake/map torque is the closed-throttle torque.
      | 2.  Shaft torque is zero.

== system lib_fuel_converter3/fuel converter <fc> no fuel at negative torque/IC Engine Model  &  Interface/ic engine model/engine torque/T_closed throttle ==
  w_APU : Inport  Port=1  LatchInput=off
  Saturation : Saturate  UpperLimit=max(fc_map_spd)*fc_spd_scale  LowerLimit=min(fc_map_spd)*fc_spd_scale  LinearizeAsGain=on
  ctt lookup : Lookup  InputValues=fc_map_spd*fc_spd_scale  OutputValues=fc_ct_trq*fc_trq_scale
  T_closed throttle : Outport  Port=1  InitialOutput=0
  wires:
  w_APU/1 -> Saturation/1
  Saturation/1 -> ctt lookup/1
  ctt lookup/1 -> T_closed throttle/1

== system lib_fuel_converter3/fuel converter <fc> no fuel at negative torque/IC Engine Model  &  Interface/ic engine model/engine torque/T_max ==
  w_APU : Inport  Port=1  LatchInput=off
  Saturation1 : Saturate  UpperLimit=max(fc_map_spd)*fc_spd_scale  LowerLimit=min(fc_map_spd)*fc_spd_scale  LinearizeAsGain=on
  max_torque lookup : Lookup  InputValues=fc_map_spd*fc_spd_scale  OutputValues=fc_max_trq*fc_trq_scale
  T_max : Outport  Port=1  InitialOutput=0
  tag scope: engine_speed=scoped
  wires:
  Saturation1/1 -> [engine_speed], max_torque lookup/1
  max_torque lookup/1 -> T_max/1
  w_APU/1 -> Saturation1/1

== system lib_fuel_converter3/fuel converter <fc> no fuel at negative torque/IC Engine Model  &  Interface/ic engine model/engine torque/effect of inertia (Nm) ==
  engine spd (rad/s) : Inport  Port=1  LatchInput=off
  >=0 : Saturate  UpperLimit=inf  LowerLimit=0  LinearizeAsGain=on
  Block NOTES : Subsystem
      settings: RTWFcnNameOpts=Auto  RTWFileNameOpts=Auto
      mask Display: disp('Block\nNOTES')
  Clock : Clock
      settings: DisplayTime=off  Decimation=10
  Constant : Constant  Orientation=left  Value=fc_inertia
  Constant1 : Constant  Value=max(fc_max_trq)*fc_trq_scale
  Constant2 : Constant  Orientation=left  Value=0.01
  Memory : Memory  X0=-0.1  InheritSampleTime=off
      settings: RTWStateStorageClass=Auto
  Memory1 : Memory  X0=vc_idle_spd*vc_key_on(1,2)  InheritSampleTime=off
      settings: RTWStateStorageClass=Auto
  Memory2 : Memory  X0=0  InheritSampleTime=off
      settings: RTWStateStorageClass=Auto
  MinMax : MinMax  Function=min  Inputs=2
  Product : Product  Inputs=2  Multiplication=Element-wise(.*)  SaturateOnIntegerOverflow=on
  Product1 : Product  Inputs=*/*  Multiplication=Element-wise(.*)  SaturateOnIntegerOverflow=on
  Relational : RelationalOperator  Operator=>
  Sum : Sum  Inputs=+-  SaturateOnIntegerOverflow=on
  Sum1 : Sum  Inputs=+-  SaturateOnIntegerOverflow=on
  Sum2 : Sum  Inputs=-+  SaturateOnIntegerOverflow=on
  Switch : Switch  Threshold=eps
  engine inertia as a function of total vehicle inertia (generous approximation) : Subsystem  Orientation=down
      settings: RTWFcnNameOpts=Auto  RTWFileNameOpts=Auto
  (Nm) : Outport  Port=1  InitialOutput=0
  wires:
  engine spd (rad/s)/1 -> Sum/1, Memory1/1
  Constant2/1 -> Relational/2
  Sum2/1 -> Relational/1
  >=0/1 -> Switch/1
  Relational/1 -> Memory2/1
  Memory2/1 -> Switch/2
  Clock/1 -> Sum1/1, Memory/1
  Memory/1 -> Sum1/2
  Constant/1 -> Product1/3
  Sum1/1 -> Product1/2
  Switch/1 -> Product1/1
  [mpha] -> Sum2/1
  [cyc_mph_r] -> Sum2/2
  MinMax/1 -> (Nm)/1
  Product1/1 -> MinMax/2
  engine inertia as a function of total vehicle inertia (generous approximation)/1(Out1) -> Product/1
  Constant1/1 -> Product/2
  Product/1 -> MinMax/1
  Memory1/1 -> Sum/2
  Sum/1 -> Switch/3, >=0/1

== system lib_fuel_converter3/fuel converter <fc> no fuel at negative torque/IC Engine Model  &  Interface/ic engine model/engine torque/enhancedToWorkspace ==
  In1 : Inport  Port=1  LatchInput=off
  To Workspace : ToWorkspace  VariableName=fc_decceleration_cmd  SampleTime=-1  SaveFormat=Array
  wires:
  In1/1 -> To Workspace/1

== system lib_fuel_converter3/fuel converter <fc> no fuel at negative torque/IC Engine Model  &  Interface/ic engine model/fuel use and EO emis no fuel used at negative torque/Block NOTES ==
  note: This block determines actual fuel use and engine-out emissions
      | given the fully hot values and the engine coolant temperature.
      | The correlations used here were developed at NREL using
      | FTP data collected under subcontract by JDM & Associates.
      | Note: PM hot/cold relation assumed same as HC
